simulink model "Expriment_Gaze"  (R2014a)
settings: Solver=FixedStepDiscrete  SolverMode=SingleTasking  StartTime=0.0  StopTime=inf  FixedStep=0.01  RelTol=1e-3
PostLoadFcn:
  | h_RPStest = RPStest;
model workspace (MAT data in the model file):
  gtest = 0
undefined symbols (not defined in the file or in its folder): avert, avert_freq_factor, avert_gaze_dirs_chance, avert_gaze_duration_factor, avert_head_frequency_factor, avert_head_speed, BML, BML1, BML2, bmlsL, bmlsM, bodyBusyFlag, clock, emotion_amount_factor, faceBusyFlag, fileID, GAZE_WIN, gazing, mut_freq_factor, mutual_gaze_duration_factor, P, pose_cat_chance, pose_chanc_factor, pose_chance_factor, pose_frequency_factor, pose_lean, pose_lean_flag, pose_speed, pose_twitch, pr, serial, STATE_BEFORE, STATE_GO, STATE_OVER, STATE_READY, Stateflow
libraries: simulink x24, instrumentlib x6, lib_affectiveChar_behavior x3, realtime_pacer_lib x2, lib_affectiveChar_input x1
(part 3 of 7)

== matlab function Expriment_Gaze/EmotionSubsystem/calculateValenceArousal/LEHN_VA_Emo ==
  data: V input; e output double size=1; A input double
function e = fcn(V, A)

aVarTruthTableCondition_1 = false;
aVarTruthTableCondition_2 = false;
aVarTruthTableCondition_3 = false;
aVarTruthTableCondition_4 = false;
aVarTruthTableCondition_5 = false;
aVarTruthTableCondition_6 = false;
aVarTruthTableCondition_7 = false;
aVarTruthTableCondition_8 = false;


% 7-happy  2,1

aVarTruthTableCondition_1 = logical(V>20 && A<40 && A>20);

% 8-ex  1,2 AND 2,2

aVarTruthTableCondition_2 = logical(V>0 && A>40);

% 4-fear  -1,2 AND -2,2

aVarTruthTableCondition_3 = logical(V<0 && A>40);

% 3-frust  -2,1

aVarTruthTableCondition_4 = logical(V<-20 && A<40 && A>20);

% 6-idle  2,-1

aVarTruthTableCondition_5 = logical(V>20 && A<-20 && A>-40);

% 5-calm  1,-2 AND 2,-2

aVarTruthTableCondition_6 = logical(V>0 && A<-40);

% 1-bored  -1,-2 AND -2,-2

aVarTruthTableCondition_7 = logical(V<0 && A<-40);

% 2-sad  -2,-1

aVarTruthTableCondition_8 = logical(V<-20 && A<-20 && A>-40);

if (aVarTruthTableCondition_1)
    aFcnTruthTableAction_1();
elseif (aVarTruthTableCondition_2)
    aFcnTruthTableAction_2();
elseif (aVarTruthTableCondition_3)
    aFcnTruthTableAction_3();
elseif (aVarTruthTableCondition_4)
    aFcnTruthTableAction_4();
elseif (aVarTruthTableCondition_5)
    aFcnTruthTableAction_5();
elseif (aVarTruthTableCondition_6)
    aFcnTruthTableAction_6();
elseif (aVarTruthTableCondition_7)
    aFcnTruthTableAction_7();
elseif (aVarTruthTableCondition_8)
    aFcnTruthTableAction_8();
else % Default
    aFcnTruthTableAction_5();
end

function aFcnTruthTableAction_1()

% happy

e=7;

function aFcnTruthTableAction_2()

% excited

e=8;

function aFcnTruthTableAction_3()

% fear

e=4;

function aFcnTruthTableAction_4()

% frustration

e=3;

function aFcnTruthTableAction_5()

% idle

e=6;

function aFcnTruthTableAction_6()

% contempt

e=5;

function aFcnTruthTableAction_7()

% bored

e=1;

function aFcnTruthTableAction_8()

% sad

e=2;

== matlab function Expriment_Gaze/EmotionSubsystem/calculateValenceArousal/LEHN_A ==
  data: a2 output double size=1; a1 input double size=1
function a2 = fcn(a1)

aVarTruthTableCondition_1 = false;
aVarTruthTableCondition_2 = false;



aVarTruthTableCondition_1 = logical(a1>25);


aVarTruthTableCondition_2 = logical(a1<-25);

if (aVarTruthTableCondition_1)
    aFcnTruthTableAction_1();
elseif (aVarTruthTableCondition_2)
    aFcnTruthTableAction_2();
else % Default
    aFcnTruthTableAction_3();
end

function aFcnTruthTableAction_1()


a2=a1;

function aFcnTruthTableAction_2()


a2=a1;

function aFcnTruthTableAction_3()


a2=0;

== matlab function Expriment_Gaze/poseInputArray/makePoseArray ==
  data: r1 input; y output double size=[1,6]; r2 input; r3 input; r4 input; r5 input; r6 input
function y = fcn(r1,r2,r3,r4,r5,r6)
%#codegen
y=[0,0,0,0,0,0];
y(:,1) = floor(r1);
y(:,2) = floor(r2);
y(:,3) = floor(r3);
y(:,4) = floor(r4);
y(:,5) = floor(r5);
y(:,6) = floor(r6);

== matlab function Expriment_Gaze/EmotionSubsystem/calculateValenceArousal/HEHN plot ==
  data: v input; a input
function fcn(v,a)
%coder.extrinsic to bypass code generation
coder.extrinsic('fscanf')
coder.extrinsic('get_param');
% coder.extrinsic('importdata');

currentTime=get_param('Expriment_FacialExpr','SimulationTime');%use name of simulink proj

A = [v;a;currentTime];
fileID = fopen('HEHN_VA_table.txt','a');
fprintf(fileID,'%0.1f,%0.1f,%0.1f\r\n',A);
fclose(fileID);

% matrix = importdata('HEHN_VA_table.txt',','); 
% tri = delaunay(matrix(:,1),matrix(:,2));
% trisurf(tri,matrix(:,1),matrix(:,2),matrix(:,3))
% shading interp
% colorbar

%-----------------------------------------
% fileID = fopen('HEHN_VA_table.txt','r');
% formatSpec = '%1f\r %1f\r %1f\r\n';
% sizeA = [3 Inf];
% A = fscanf(fileID,formatSpec,sizeA)
% % A = A'
% fclose(fileID);

% x = zeros(100,2);y = zeros(100,2);
% filename = 'HEHN_VA_table.txt';
% delimiterIn = ' ';
% headerlinesIn = 1;
% A = importdata(filename,delimiterIn,headerlinesIn);

% fileID=fopen('HEHN_VA_table4.txt');
% s=textscan(fileID,'%d %d %d','headerlines',23);
% fclose(fileID);
% x=s{1}

== matlab function Expriment_Gaze/EmotionSubsystem/calculateValenceArousal/LEHN plot ==
  data: v input; a input
function fcn(v,a)
%coder.extrinsic to bypass code generation
coder.extrinsic('fscanf')
coder.extrinsic('get_param');
% coder.extrinsic('importdata');

currentTime=get_param('Expriment_FacialExpr','SimulationTime');%use name of simulink proj

A = [v;a;currentTime];

fileID = fopen('LEHN_VA_table.txt','a');
fprintf(fileID,'%0.1f,%0.1f,%0.1f\r\n',A);
fclose(fileID);

%use the following to draw the plot
%tmp_data = importdata('HEHN_VA_table.txt',','); 
%no need: x=tmp_data(:,1);y=tmp_data(:,2);z=tmp_data(:,3)
%matrix=tmp_data
%tri = delaunay(matrix(:,1),matrix(:,2));
%trisurf(tri,matrix(:,1),matrix(:,2),matrix(:,3))
%shading interp

%-----------------------------------------
% fileID = fopen('HEHN_VA_table.txt','r');
% formatSpec = '%1f\r %1f\r %1f\r\n';
% sizeA = [3 Inf];
% A = fscanf(fileID,formatSpec,sizeA)
% % A = A'
% fclose(fileID);

% x = zeros(100,2);y = zeros(100,2);
% filename = 'HEHN_VA_table.txt';
% delimiterIn = ' ';
% headerlinesIn = 1;
% A = importdata(filename,delimiterIn,headerlinesIn);

% fileID=fopen('HEHN_VA_table4.txt');
% s=textscan(fileID,'%d %d %d','headerlines',23);
% fclose(fileID);
% x=s{1}

== matlab function Expriment_Gaze/EmotionSubsystem/calculateValenceArousal/LELN plot ==
  data: v input; a input
function fcn(v,a)
%coder.extrinsic to bypass code generation
coder.extrinsic('fscanf')
coder.extrinsic('get_param');
% coder.extrinsic('importdata');

currentTime=get_param('Expriment_FacialExpr','SimulationTime');%use name of simulink proj

A = [v;a;currentTime];

fileID = fopen('LELN_VA_table.txt','a');
fprintf(fileID,'%0.1f,%0.1f,%0.1f\r\n',A);
fclose(fileID);

%use the following to draw the plot
%matrix = importdata('HEHN_VA_table.txt',','); 
%tri = delaunay(matrix(:,1),matrix(:,2));
%trisurf(tri,matrix(:,1),matrix(:,2),matrix(:,3))
%shading interp
%colorbar
%-----------------------------------------
% fileID = fopen('HEHN_VA_table.txt','r');
% formatSpec = '%1f\r %1f\r %1f\r\n';
% sizeA = [3 Inf];
% A = fscanf(fileID,formatSpec,sizeA)
% % A = A'
% fclose(fileID);

% x = zeros(100,2);y = zeros(100,2);
% filename = 'HEHN_VA_table.txt';
% delimiterIn = ' ';
% headerlinesIn = 1;
% A = importdata(filename,delimiterIn,headerlinesIn);

% fileID=fopen('HEHN_VA_table4.txt');
% s=textscan(fileID,'%d %d %d','headerlines',23);
% fclose(fileID);
% x=s{1}

== matlab function Expriment_Gaze/EmotionSubsystem/calculateValenceArousal/HELN_V ==
  data: v2 output double size=1; v1 input double size=1
function v2 = fcn(v1)

aVarTruthTableCondition_1 = false;
aVarTruthTableCondition_2 = false;



aVarTruthTableCondition_1 = logical(v1>10);


aVarTruthTableCondition_2 = logical(v1<-10);

if (aVarTruthTableCondition_1)
    aFcnTruthTableAction_1();
elseif (aVarTruthTableCondition_2)
    aFcnTruthTableAction_2();
else % Default
    aFcnTruthTableAction_3();
end

function aFcnTruthTableAction_1()


v2=v1;

function aFcnTruthTableAction_2()


v2=v1;

function aFcnTruthTableAction_3()


v2=0;

== matlab function Expriment_Gaze/EmotionSubsystem/calculateValenceArousal/LELN_V ==
  data: v2 output double size=1; v1 input double size=1
function v2 = fcn(v1)

aVarTruthTableCondition_1 = false;
aVarTruthTableCondition_2 = false;



aVarTruthTableCondition_1 = logical(v1>25);


aVarTruthTableCondition_2 = logical(v1<-25);

if (aVarTruthTableCondition_1)
    aFcnTruthTableAction_1();
elseif (aVarTruthTableCondition_2)
    aFcnTruthTableAction_2();
else % Default
    aFcnTruthTableAction_3();
end

function aFcnTruthTableAction_1()


v2=v1;

function aFcnTruthTableAction_2()


v2=v1;

function aFcnTruthTableAction_3()


v2=0;
